simulink model "untitled1"  (R2023a)
settings: Solver=VariableStepAuto  StartTime=0.0  StopTime=10.0  RelTol=1e-3
libraries: fl_lib x8
settings Model: Creator=Aguer  LastModifiedBy=Aguer

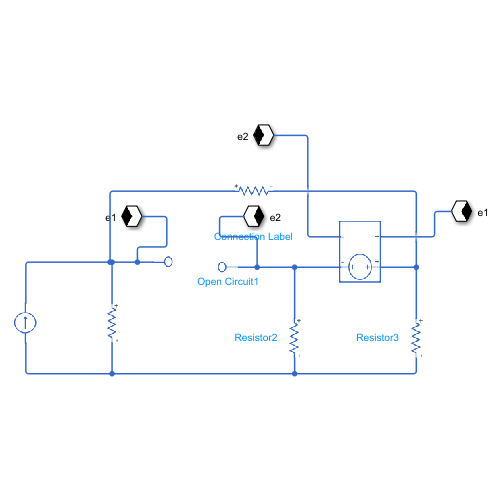
[thumbnail: Simulink's stored preview of the top-level diagram]
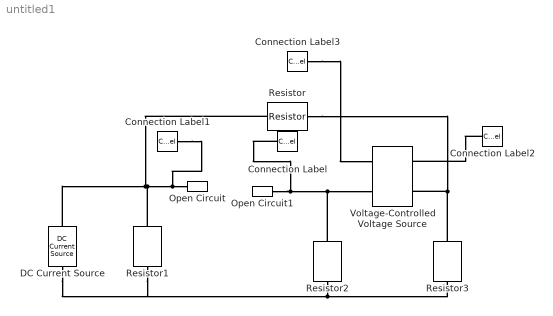
== system untitled1 ==
  Connection Label : ConnectionLabel  Label=e2
  Connection Label1 : ConnectionLabel  Label=e1
  Connection Label2 : ConnectionLabel  Label=e1
  Connection Label3 : ConnectionLabel  Label=e2
  DC Current Source : fl_lib/Electrical/Electrical Sources/DC Current Source  i0=1 A
      settings: InternalSimscapePortConfiguration="{\"Bottom\":[],\"Left\":[{\"id\":\"p\",\"label\":\"\",\"type\":\"foundation.electrical.electrical\"}],\"Right\":[{\"id\":\"n\",\"label\":\"\",\"type\":\"foundation.electrical.electrical\"}],\"Top\":[]}"
  Open Circuit : fl_lib/Electrical/Electrical Elements/Open Circuit  v_specify=off  v_priority=None  v=0 V  v_nominal_specify=off  v_nominal_unit=V  v_nominal_value=1
  Open Circuit1 : fl_lib/Electrical/Electrical Elements/Open Circuit  v_specify=off  v_priority=None  v=0 V  v_nominal_specify=off  v_nominal_unit=V  v_nominal_value=1
  Resistor{,1..3} (4 alike) : fl_lib/Electrical/Electrical Elements/Resistor  R=1 Ohm  i_specify=off  i_priority=None  i=0 A  i_nominal_specify=off  i_nominal_unit=A  i_nominal_value=1  v_specify=off  v_priority=None  v=0 V  v_nominal_specify=off  v_nominal_unit=V  v_nominal_value=1
  Voltage-Controlled Voltage Source : fl_lib/Electrical/Electrical Sources/Voltage-Controlled Voltage Source  K=1  v1_specify=off  v1_priority=None  v1=0 V  v1_nominal_specify=off  v1_nominal_unit=V  v1_nominal_value=1  v2_specify=off  v2_priority=None  v2=0 V  v2_nominal_specify=off  v2_nominal_unit=V  v2_nominal_value=1
      settings: InternalSimscapePortConfiguration="{\"Bottom\":[],\"Left\":[{\"id\":\"p1\",\"label\":\"+\",\"type\":\"foundation.electrical.electrical\"},{\"id\":\"p2\",\"label\":\"+\",\"type\":\"foundation.electrical.electrical\"}],\"Right\":[{\"id\":\"n1\",\"label\":\"-\",\"type\":\"foundation.electrical.electrical\"},{\"id\":\"n2\",\"label\":\"-\",\"type\":\"foundation.electrical.electrical\"}],\"Top\":[]}"
  connections:
  Resistor1/LConn1 -- DC Current Source/LConn1 -- Resistor/LConn1 -- Connection Label1/LConn1 -- Open Circuit/LConn1
  Open Circuit1/LConn1 -- Connection Label/LConn1 -- Resistor2/LConn1 -- Voltage-Controlled Voltage Source/RConn2
  Resistor/RConn1 -- Resistor3/LConn1 -- Voltage-Controlled Voltage Source/LConn2
  Resistor2/RConn1 -- DC Current Source/RConn1 -- Resistor1/RConn1 -- Resistor3/RConn1
  Connection Label2/LConn1 -- Voltage-Controlled Voltage Source/LConn1
  Connection Label3/LConn1 -- Voltage-Controlled Voltage Source/RConn1
